simulink model "mazeRunner"  (R2023a)
settings: Solver=FixedStepDiscrete  StartTime=0.0  StopTime=300  FixedStep=0.01  RelTol=1e-3
values from neighbouring files (symbols this model uses):
  axleLength = 0.136    [robotParameters.m]
  maxV = (160/30)*pi*wheelR    (= 0.519409985394)    [robotParameters.m]
  ticksPerRot = 20    [robotParameters.m]
  wheelR = 0.031    [robotParameters.m]
undefined symbols (not defined in the file or in its folder): InputPWM, WheelSpeed
libraries: mobileRoboticsTrainingLib x10, slpidlib x2, simulink x1
settings Model: NumberOfSteps=10  Creator=dower  LastModifiedBy=starl
settings DebuggingCC: UnderSpecifiedDimensionMsg=warning

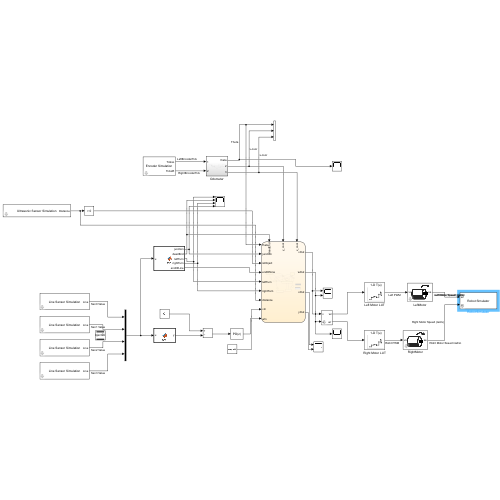
[thumbnail: Simulink's stored preview of the top-level diagram]
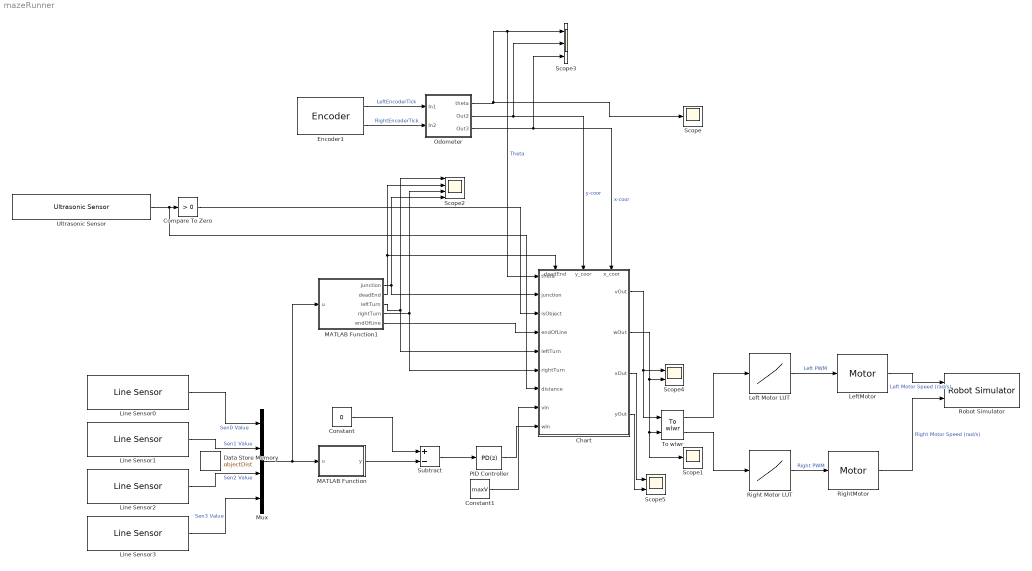
== system mazeRunner ==
  Chart : Stateflow chart  TreatAsAtomicUnit=on
      settings: PortSchema="{\"entries\":[{\"content\":{\"sides\":[{\"content\":{\"connectorIds\":[\"In10\",\"In11\",\"In12\",\"In6\",\"In4\",\"In5\",\"In7\",\"In8\",\"In9\"]},\"type\":\"ConnectorPlacement.EquallySpacedRectSide\",\"uuid\":\"57a3dc3c-5330-4212-9af6-f313022488fd\"},{\"content\":{\"connectorIds\":[\"Out1\",\"Out2\",\"Out3\",\"Out4\"],\"side\":\"RIGHT\"},\"type\":\"ConnectorPlacement.EquallySpacedRectSide\",\"uuid\":\"1070cbf7-6ba4-437e-a2a0-cd8b795bb269\"},{\"content\":{\"connectorIds\":[\"In1\",\"In2\",\"In3\"],\"side\":\"TOP\"},\"type\":\"ConnectorPlacement.EquallySpacedRectSide\",\"uuid\":\"ba30032c-ab7b-4e9d-8967-1a7a6a7ac690\"}]},\"type\":\"ConnectorPlacement.EquallySpacedConnector\",\"uuid\":\"77aefb05-3ccd-4ebf-8659-83851d1b6a76\"}],\"packageUris\":[\"http://schema.mathworks.com/mf0/Connector/R2020b\"],\"version\":\"1.0\"}"
  Compare To Zero : simulink/Logic and Bit Operations/Compare To Zero  relop=>  OutDataTypeStr=boolean
  Constant : Constant  Value=0
  Constant1 : Constant  Value=maxV
  Data Store Memory : DataStoreMemory  DataStoreName=objectDist  WriteAfterWriteMsg=warning  ShowAdditionalParam=off
  Encoder1 : mobileRoboticsTrainingLib/Encoder  axleLength=axleLength  wheelR=wheelR  ticksPerRot=ticksPerRot
      settings: SourceProductName=Mobile Robotics Training Library
  Left Motor LUT : Lookup_n-D  NumberOfTableDimensions=1  BreakpointsForDimension1=WheelSpeed  Table=InputPWM  InterpMethod=Nearest  ExtrapMethod=Clip  InternalRulePriority=Speed  RndMeth=Simplest
  LeftMotor : mobileRoboticsTrainingLib/Motor  motorPlant=wheelMotorModel  sensorType=Speed
      settings: SourceProductName=Mobile Robotics Training Library
  Line Sensor0 : mobileRoboticsTrainingLib/Line Sensor  mapVariable=mapForSim  envVal=2800  lineVal=2900  sensOff=[0.0643 0.0354]
      settings: SourceProductName=Mobile Robotics Training Library
  Line Sensor1 : mobileRoboticsTrainingLib/Line Sensor  mapVariable=mapForSim  envVal=2800  lineVal=2900  sensOff=[0.0675 0.005]
      settings: SourceProductName=Mobile Robotics Training Library
  Line Sensor2 : mobileRoboticsTrainingLib/Line Sensor  mapVariable=mapForSim  envVal=2800  lineVal=2900  sensOff=[0.0675 -0.005]
      settings: SourceProductName=Mobile Robotics Training Library
  Line Sensor3 : mobileRoboticsTrainingLib/Line Sensor  mapVariable=mapForSim  envVal=2800  lineVal=2900  sensOff=[0.0643 -0.0354]
      settings: SourceProductName=Mobile Robotics Training Library
  MATLAB Function : MATLAB Function  TreatAsAtomicUnit=on
  MATLAB Function1 : MATLAB Function  TreatAsAtomicUnit=on
  Mux : Mux
  Odometer : Subsystem
  PID Controller : slpidlib/PID Controller  Controller=PD  Form=Parallel  TimeDomain=Discrete-time  UseExternalTs=off  SampleTime=-1  IntegratorMethod=Forward Euler  FilterMethod=Forward Euler  ControllerParametersSource=internal  P=10  I=1  UseKiTs=off  D=10e-5  N=100  UseFilter=on  TunerSelectOption=Frequency Response Based  InitialConditionSource=internal  InitialConditionForIntegrator=0  InitialConditionForFilter=0  DifferentiatorICPrevScaledInput=0  ExternalReset=none  TrackingMode=off  Kt=1  LimitOutput=off  SatLimitsSource=internal  UpperSaturationLimit=inf  LowerSaturationLimit=-inf  LinearizeAsGain=on  AntiWindupMode=none  Kb=1  LimitIntegrator=off  UpperIntegratorSaturationLimit=inf  LowerIntegratorSaturationLimit=-inf  POutMin=[]  POutMax=[]  IOutMin=[]  IOutMax=[]  DOutMin=[]  DOutMax=[]  NOutMin=[]  NOutMax=[]  SumOutMin=[]  SumOutMax=[]  SaturationOutMin=[]  SaturationOutMax=[]  PParamMin=[]  PParamMax=[]  IParamMin=[]  IParamMax=[]  DParamMin=[]  DParamMax=[]  NParamMin=[]  NParamMax=[]  KbParamMin=[]  KbParamMax=[]  KtParamMin=[]  KtParamMax=[]  KbOutMin=[]  KbOutMax=[]  KtOutMin=[]  KtOutMax=[]  IntegratorOutMin=[]  IntegratorOutMax=[]  FilterOutMin=[]  FilterOutMax=[]  SumI1OutMin=[]  SumI1OutMax=[]  SumI2OutMin=[]  SumI2OutMax=[]  SumI3OutMin=[]  SumI3OutMax=[]  SumI4OutMin=[]  SumI4OutMax=[]  SumDOutMin=[]  SumDOutMax=[]  DifferentiatorOutMin=[]  DifferentiatorOutMax=[]  FilterDiffOutCoefMin=[]  FilterDiffOutCoefMax=[]  ReciprocalOutMin=[]  ReciprocalOutMax=[]  SumDenOutMin=[]  SumDenOutMax=[]  SumNumOutMin=[]  SumNumOutMax=[]  DivideOutMin=[]  DivideOutMax=[]  UdiffTsProdOutMin=[]  UdiffTsProdOutMax=[]  NTsProdOutMin=[]  NTsProdOutMax=[]  UintegralTsProdOutMin=[]  UintegralTsProdOutMax=[]  UngainTsProdOutMin=[]  UngainTsProdOutMax=[]  ClampingZeroOutDataTypeStr=Inherit: Inherit via back propagation  ClampingZeroOutMin=[]  ClampingZeroOutMax=[]  FilterDenConstantOutDataTypeStr=Inherit: Inherit via back propagation  FilterDenConstantOutMin=[]  FilterDenConstantOutMax=[]  PCopyOutDataTypeStr=Inherit: Inherit via back propagation  PCopyOutMin=[]  PCopyOutMax=[]  NCopyOutDataTypeStr=Inherit: Inherit via back propagation  NCopyOutMin=[]  NCopyOutMax=[]  IntegratorContinuousStateAttributes=''  IntegratorStateMustResolveToSignalObject=off  IntegratorRTWStateStorageClass=Auto  FilterContinuousStateAttributes=''  FilterStateMustResolveToSignalObject=off  FilterRTWStateStorageClass=Auto  ParallelPVariant=InternalParameters  IdealPVariant=Disabled  IVariant=Disabled  DVariant=InternalParameters  IntegratorVariant=Disabled  SatVariant=Disabled  AWVariant=Disabled  PCopyVariant=Disabled  TRVariant=Disabled  FdbkBlocksVariant=Forward  IdealPFdbkVariant=Disabled  SatFdbkVariant=Disabled  DerivativeFilterVariant=ForwardEulerFilter  NVariant=InternalParameters  NCopyVariant=Disabled  FilterICVariant=InternalICsFilter  IntegratorICVariant=Disabled  ExternalResetVariant=Disabled  TRSumVariant=Passthrough  SumFdbkVariant=Disabled  SumVariant=Sum_PD  TsampFilterVariant=InternalTs  TsampNgainVariant=Passthrough  TsampIntegralVariant=Disabled_SignalSpec  ExternalSaturationOutDataTypeStr=Inherit: Same as second input
  Right Motor LUT : Lookup_n-D  NumberOfTableDimensions=1  BreakpointsForDimension1=WheelSpeed  Table=InputPWM  InterpMethod=Nearest  ExtrapMethod=Clip  InternalRulePriority=Speed  RndMeth=Simplest
  RightMotor : mobileRoboticsTrainingLib/Motor  motorPlant=wheelMotorModel  sensorType=Speed
      settings: SourceProductName=Mobile Robotics Training Library
  Robot Simulator : mobileRoboticsTrainingLib/Robot Simulator  Priority=99  mapVar=mapForSim  startX=1.2431  startY=3.095  startTheta=0  axleLength=axleLength  wheelR=wheelR
  Scope : Scope
  Scope1 : Scope
  Scope2 : Scope  NumInputPorts=4
  Scope3 : Scope  NumInputPorts=3
  Scope4 : Scope  NumInputPorts=2
  Scope5 : Scope  NumInputPorts=2
  Subtract : Sum  Inputs=+-
  To wlwr : mobileRoboticsTrainingLib/To wlwr  axleLength=0.1  wheelR=0.05
  Ultrasonic Sensor : mobileRoboticsTrainingLib/Ultrasonic Sensor  mapVar=mapForSim  maxSenRange=2  minSenRange=0.02  senRes=0.01  sensOff=[0 0]
      settings: SourceProductName=Mobile Robotics Training Library
  wires:
  Line Sensor1/1 -> Mux/2  "Sen1 Value"
  Subtract/1 -> PID Controller/1
  Right Motor LUT/1 -> RightMotor/1  "Right PWM"
  Constant/1 -> Subtract/1
  LeftMotor/1 -> Robot Simulator/1  "Left Motor Speed (rad/s)"
  Line Sensor0/1 -> Mux/1  "Sen0 Value"
  Mux/1 -> MATLAB Function1/1(u), MATLAB Function/1(u)
  Line Sensor2/1 -> Mux/3  "Sen2 Value"
  Left Motor LUT/1 -> LeftMotor/1  "Left PWM"
  Line Sensor3/1 -> Mux/4  "Sen3 Value"
  To wlwr/1 -> Left Motor LUT/1
  To wlwr/2 -> Right Motor LUT/1
  RightMotor/1 -> Robot Simulator/2  "Right Motor Speed (rad/s)"
  MATLAB Function/1(y) -> Subtract/2
  Ultrasonic Sensor/1 -> Chart/7(distance), Compare To Zero/1
  Compare To Zero/1 -> Chart/12(isObject)
  PID Controller/1 -> Chart/9(wIn)
  MATLAB Function1/1(junction) -> Scope2/4, Chart/11(junction)
  Chart/1(vOut) -> Scope4/1, To wlwr/1
  Chart/2(wOut) -> Scope1/1, To wlwr/2, Scope4/2
  Odometer/1(theta) -> Scope3/1, Chart/10(theta), Scope/1  "Theta"
  Odometer/2(Out2) -> Chart/2(y_coor), Scope3/2  "y-coor"
  Encoder1/1 -> Odometer/1(In1)  "LeftEncoderTick"
  Encoder1/2 -> Odometer/2(In2)  "RightEncoderTick"
  Odometer/3(Out3) -> Chart/3(x_coor), Scope3/3  "x-coor"
  MATLAB Function1/2(deadEnd) -> Chart/1(deadEnd), Scope2/2
  Constant1/1 -> Chart/8(vIn)
  MATLAB Function1/3(leftTurn) -> Scope2/1, Chart/4(leftTurn)
  MATLAB Function1/4(rightTurn) -> Chart/5(rightTurn), Scope2/3
  MATLAB Function1/5(endOfLine) -> Chart/6(endOfLine)
  Chart/3(xOut) -> Scope5/1
  Chart/4(yOut) -> Scope5/2

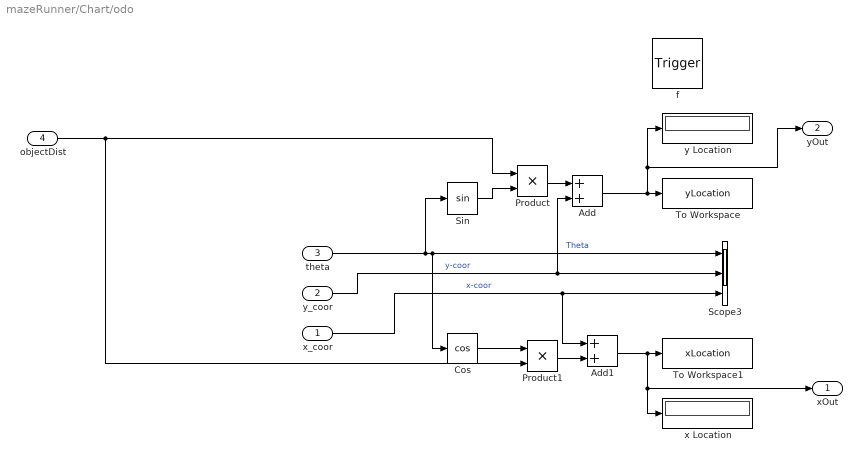
== system mazeRunner/Chart/odo ==
  x_coor : Inport  OutDataTypeStr=double  PortDimensions=1
  y_coor : Inport  Port=2  OutDataTypeStr=double  PortDimensions=1
  theta : Inport  Port=3  OutDataTypeStr=double  PortDimensions=1
  objectDist : Inport  Port=4  OutDataTypeStr=double  PortDimensions=1
  f : TriggerPort  TriggerType=function-call  VariantControl=(inherit)
      settings: CopyFcn=Stateflow.SLINSF.SimulinkMan.removeBlockPreDeleteFcn  PreDeleteFcn=Stateflow.SLINSF.SimulinkMan.unsafePredeleteFcn
  Add : Sum
  Add1 : Sum
  Cos : Trigonometry  Operator=cos
  Product : Product
  Product1 : Product
  Scope3 : Scope  NumInputPorts=3
  Sin : Trigonometry
  To Workspace : ToWorkspace  VariableName=yLocation  SaveFormat=Timeseries  SampleTime=-1
  To Workspace1 : ToWorkspace  VariableName=xLocation  SaveFormat=Timeseries  SampleTime=-1
  x Location : Display
  y Location : Display
  xOut : Outport
  yOut : Outport  Port=2
  wires:
  Add1/1 -> xOut/1, x Location/1, To Workspace1/1
  objectDist/1 -> Product1/2, Product/1
  y_coor/1 -> Add/2, Scope3/2  "y-coor"
  Sin/1 -> Product/2
  Product1/1 -> Add1/2
  Cos/1 -> Product1/1
  theta/1 -> Cos/1, Scope3/1, Sin/1  "Theta"
  Product/1 -> Add/1
  x_coor/1 -> Add1/1, Scope3/3  "x-coor"
  Add/1 -> yOut/1, y Location/1, To Workspace/1

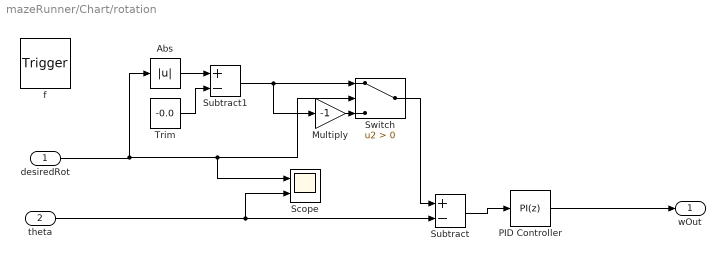
== system mazeRunner/Chart/rotation ==
  desiredRot : Inport  OutDataTypeStr=double  PortDimensions=1
  theta : Inport  Port=2  OutDataTypeStr=double  PortDimensions=1
  f : TriggerPort  TriggerType=function-call  VariantControl=(inherit)
      settings: CopyFcn=Stateflow.SLINSF.SimulinkMan.removeBlockPreDeleteFcn  PreDeleteFcn=Stateflow.SLINSF.SimulinkMan.unsafePredeleteFcn
  Abs : Abs  SaturateOnIntegerOverflow=off
  Multiply : Gain  Gain=-1
  PID Controller : slpidlib/PID Controller  Controller=PI  Form=Ideal  TimeDomain=Discrete-time  UseExternalTs=off  SampleTime=-1  IntegratorMethod=Forward Euler  FilterMethod=Forward Euler  ControllerParametersSource=internal  P=18  I=0.2  UseKiTs=off  D=0.02  N=100  UseFilter=on  TunerSelectOption=Frequency Response Based  InitialConditionSource=internal  InitialConditionForIntegrator=0  InitialConditionForFilter=0  DifferentiatorICPrevScaledInput=0  ExternalReset=none  TrackingMode=off  Kt=1  LimitOutput=on  SatLimitsSource=internal  UpperSaturationLimit=maxV  LowerSaturationLimit=-maxV  LinearizeAsGain=on  AntiWindupMode=clamping  Kb=1  LimitIntegrator=off  UpperIntegratorSaturationLimit=inf  LowerIntegratorSaturationLimit=-inf  POutMin=[]  POutMax=[]  IOutMin=[]  IOutMax=[]  DOutMin=[]  DOutMax=[]  NOutMin=[]  NOutMax=[]  SumOutMin=[]  SumOutMax=[]  SaturationOutMin=[]  SaturationOutMax=[]  PParamMin=[]  PParamMax=[]  IParamMin=[]  IParamMax=[]  DParamMin=[]  DParamMax=[]  NParamMin=[]  NParamMax=[]  KbParamMin=[]  KbParamMax=[]  KtParamMin=[]  KtParamMax=[]  KbOutMin=[]  KbOutMax=[]  KtOutMin=[]  KtOutMax=[]  IntegratorOutMin=[]  IntegratorOutMax=[]  FilterOutMin=[]  FilterOutMax=[]  SumI1OutMin=[]  SumI1OutMax=[]  SumI2OutMin=[]  SumI2OutMax=[]  SumI3OutMin=[]  SumI3OutMax=[]  SumI4OutMin=[]  SumI4OutMax=[]  SumDOutMin=[]  SumDOutMax=[]  DifferentiatorOutMin=[]  DifferentiatorOutMax=[]  FilterDiffOutCoefMin=[]  FilterDiffOutCoefMax=[]  ReciprocalOutMin=[]  ReciprocalOutMax=[]  SumDenOutMin=[]  SumDenOutMax=[]  SumNumOutMin=[]  SumNumOutMax=[]  DivideOutMin=[]  DivideOutMax=[]  UdiffTsProdOutMin=[]  UdiffTsProdOutMax=[]  NTsProdOutMin=[]  NTsProdOutMax=[]  UintegralTsProdOutMin=[]  UintegralTsProdOutMax=[]  UngainTsProdOutMin=[]  UngainTsProdOutMax=[]  ClampingZeroOutDataTypeStr=Inherit: Inherit via back propagation  ClampingZeroOutMin=[]  ClampingZeroOutMax=[]  FilterDenConstantOutDataTypeStr=Inherit: Inherit via back propagation  FilterDenConstantOutMin=[]  FilterDenConstantOutMax=[]  PCopyOutDataTypeStr=Inherit: Inherit via back propagation  PCopyOutMin=[]  PCopyOutMax=[]  NCopyOutDataTypeStr=Inherit: Inherit via back propagation  NCopyOutMin=[]  NCopyOutMax=[]  IntegratorContinuousStateAttributes=''  IntegratorStateMustResolveToSignalObject=off  IntegratorRTWStateStorageClass=Auto  FilterContinuousStateAttributes=''  FilterStateMustResolveToSignalObject=off  FilterRTWStateStorageClass=Auto  ParallelPVariant=Passthrough  IdealPVariant=InternalParameters  IVariant=InternalParameters  DVariant=Disabled  IntegratorVariant=Discrete  SatVariant=Enabled  AWVariant=DiscClampingIdeal  PCopyVariant=InternalParamsIdeal  TRVariant=Disabled  FdbkBlocksVariant=Forward  IdealPFdbkVariant=Disabled  SatFdbkVariant=Disabled  DerivativeFilterVariant=Disabled  NVariant=Disabled  NCopyVariant=Disabled_SignalSpec  FilterICVariant=Disabled  IntegratorICVariant=InternalICs  ExternalResetVariant=Disabled  TRSumVariant=Passthrough  SumFdbkVariant=Disabled  SumVariant=Sum_PI  TsampFilterVariant=InternalTs  TsampNgainVariant=Passthrough  TsampIntegralVariant=Disabled_SignalSpec  ExternalSaturationOutDataTypeStr=Inherit: Same as second input
  Scope : Scope  NumInputPorts=2
  Subtract : Sum  Inputs=+-
  Subtract1 : Sum  Inputs=+-
  Switch : Switch  Criteria=u2 > Threshold  SaturateOnIntegerOverflow=off  InputSameDT=off
  Trim : Constant  Value=-0.0
  wOut : Outport
  wires:
  PID Controller/1 -> wOut/1
  Subtract/1 -> PID Controller/1
  desiredRot/1 -> Scope/1, Switch/2, Abs/1
  Abs/1 -> Subtract1/1
  Trim/1 -> Subtract1/2
  Subtract1/1 -> Switch/1, Multiply/1
  Multiply/1 -> Switch/3
  Switch/1 -> Subtract/1
  theta/1 -> Scope/2, Subtract/2

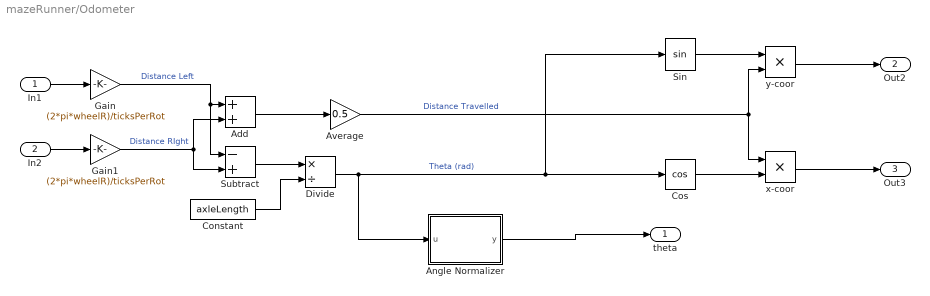
== system mazeRunner/Odometer ==
  In1 : Inport
  In2 : Inport  Port=2
  Add : Sum
  Angle Normalizer : MATLAB Function  TreatAsAtomicUnit=on
  Average : Gain  Gain=0.5
  Constant : Constant  Value=axleLength
  Cos : Trigonometry  Operator=cos  OutputSignalType=real
  Divide : Product  Inputs=*/
  Gain : Gain  Gain=(2*pi*wheelR)/ticksPerRot
  Gain1 : Gain  Gain=(2*pi*wheelR)/ticksPerRot
  Sin : Trigonometry  OutputSignalType=real
  Subtract : Sum  Inputs=-+
  x-coor : Product
  y-coor : Product
  theta : Outport
  Out2 : Outport  Port=2
  Out3 : Outport  Port=3
  wires:
  x-coor/1 -> Out3/1
  Divide/1 -> Sin/1, Cos/1, Angle Normalizer/1(u)  "Theta (rad)"
  Gain/1 -> Subtract/1, Add/1  "Distance Left"
  In1/1 -> Gain/1
  Cos/1 -> x-coor/2
  Subtract/1 -> Divide/1
  Add/1 -> Average/1
  Average/1 -> x-coor/1, y-coor/2  "Distance Travelled"
  Gain1/1 -> Add/2, Subtract/2  "Distance RIght"
  Sin/1 -> y-coor/1
  In2/1 -> Gain1/1
  Constant/1 -> Divide/2
  y-coor/1 -> Out2/1
  Angle Normalizer/1(y) -> theta/1

== matlab function mazeRunner/MATLAB Function1 ==
  data: junction output; u input; deadEnd output; leftTurn output; rightTurn output; endOfLine output
function [junction, deadEnd, leftTurn, rightTurn, endOfLine]  = fcn(u)
totalZero = 0;
deadEnd = false;
junction = false;
endOfLine = false;
leftTurn = 0;
rightTurn = 0;

for i=1:1:size(u, 1)
    if (u(i) == 2800)
        totalZero = totalZero + 1;
    end
end

if u(1, 1) == 2900 && u(4, 1) == 2900
    junction = true; %at junction, possible object

elseif u(1, 1) == 2900 && u(4, 1) == 2800
    %pause(0.05)
    if u(1, 1) == 2900 && u(4, 1) == 2900
        junction = true; %at junction, possible object
    
    else
        leftTurn = leftTurn + 1;
    end


elseif u(4, 1) == 2900 && u(1, 1) == 2800
    %pause(0.05)
    if u(1, 1) == 2900 && u(4, 1) == 2900
        junction = true; %at junction, possible object
 
    else
        rightTurn = rightTurn + 1;
    end
elseif totalZero == size(u, 1) 
    deadEnd = true; %if at deadend (no stop line, no object)
elseif totalZero == 0
    endOfLine = true;
end

== matlab function mazeRunner/MATLAB Function ==
  data: u input; y output
function y = fcn(u)
totalZero = 0;
for i=1:1:size(u, 1)
    if (u(i) == 2800)
        totalZero = totalZero + 1;
    end
end

if totalZero == 0
    y = -10;
else
    y = ((u(1)*-2)+(u(2)*-1)+(u(3)*1)+(u(4)*2))/totalZero;
end

== stateflow chart mazeRunner/Chart ==
  state RightTurn
    entry, during:
    vOut = 0.02
    desTheta = initTheta-pi/2
    wOut  = rotation(desTheta,theta)
    isRight = true
    if hasTurned == true
    hasTurned = false
    isRight = false
    end
  state LeftTurn
    entry, during:
    vOut = 0.02
    desTheta = initTheta+pi/2
    wOut  = rotation(desTheta,theta)
    isRight = false
    if hasTurned == true
    hasTurned = false
    else
    hasTurned = true
    end
  state CheckR
    after(0.1,sec)
  state Wait
  state CheckL
    after(0.1,sec)
  state initialize
    entry: hasTurned = false
    isRight = false
  state lineStopDetected
    entry, during: vOut=0.0
    wOut = 0
    initTheta = theta
  state lineFollowing
    entry, during:
    wOut = wIn
    vOut = vIn
  state [xOut,yOut] = odo(x_coor, y_coor, theta, objectDist) [function]
  state Stop
    entry: vOut = -0.005
    wOut = 0
  state wOut = rotation(desiredRot, theta) [function]
  state Start
    entry: vOut = 0
    wOut = 0
  state turnAround
    entry, during:
    vOut = 0
    desTheta = initTheta-pi
    wOut  = rotation(desTheta,theta)
    hasTurned = true
  state measureObject
    entry:  objectDist = distance
    [xOut, yOut]= odo(x_coor, y_coor, theta, objectDist)
  CheckR -> RightTurn [order 2] : [junction == false]{initTheta = theta}
  lineStopDetected -> LeftTurn [order 3] : [isRight == false && hasTurned == true && isObject == false]{initTheta = theta}
  RightTurn -> lineFollowing : after(3, sec)
  lineStopDetected -> RightTurn [order 1] : [ isObject == false]{initTheta = theta}
  LeftTurn -> lineFollowing : after(3,sec)
  Wait -> LeftTurn [order 1] : [junction == false]{initTheta = theta}
  CheckR -> lineStopDetected [order 1] : [junction == true]
  CheckR -> lineFollowing [order 3] : [goHome == true]{wOut = 0, vOut = vIn}
  lineFollowing -> CheckR [order 2] : [rightTurn == 1 && junction == false]
  Wait -> lineStopDetected [order 2] : [junction == true]
  Wait -> lineFollowing [order 3] : [goHome == true]{wOut = 0, vOut = vIn}
  CheckL -> Wait : after(0.005,sec)
  (default) -> initialize
  lineFollowing -> CheckL [order 1] : [leftTurn == 1 && junction == false]
  initialize -> lineFollowing : [true]
  lineFollowing -> lineStopDetected [order 4] : [junction == true]
  lineStopDetected -> Start [order 2] : [isObject == true]
  lineFollowing -> turnAround [order 5] : [endOfLine == true]{goHome = true, initTheta = theta}
  turnAround -> lineFollowing : after(3,sec)
  lineFollowing -> Stop [order 3] : [deadEnd == true]
  Stop -> turnAround : [deadEnd == false]{initTheta = theta}
  Start -> measureObject : after(1,sec)
  measureObject -> turnAround : [objectDist>0]{initTheta = theta}
  data: x_coor function_input double size=1; y_coor function_input double size=1; theta function_input double size=1; xOut function_output; yOut function_output; objectDist function_input double size=1; desiredRot function_input double size=1; wOut function_output; theta function_input double size=1; deadEnd input; y_coor input; x_coor input; leftTurn input; rightTurn input; endOfLine input; distance input; vOut output; wOut output; vIn input; wIn input; theta input; desTheta local; junction input; hasTurned local; objectDist local; initTheta local; isRight local; isObject input; goHome local; xOut output; yOut output

== matlab function mazeRunner/Odometer/Angle Normalizer ==
  data: u input; y output
function y = fcn(u)
if u>2*pi
    y = mod(u,2*pi);
else
    y = u;
end
